simulink model "io305"  (Simulink 6.0)
settings: Solver=ode5  StartTime=0.0  StopTime=5  RelTol=1e-3
libraries: xpcdiamondlib x2
settings Model: Creator=ekbas  LastModifiedBy=ekbas  ExtModeArmWhenConnect=off  BufferReuse=off  ProdHWDeviceType=Specified
settings DataIOCC: SaveFormat=Structure  SignalLoggingName=sigsOut
settings OptimizationCC: OptimizeBlockIOStorage=off  BufferReuse=off  LocalBlockOutputs=off
settings DebuggingCC: CheckExecutionContextPreStartOutputMsg=on  CheckExecutionContextRuntimeOutputMsg=on  SolverPrmCheckMsg=none
settings HardwareCC: ProdHWDeviceType=Specified  TargetHWDeviceType=32-bit Generic  ProdEqTarget=off
settings RTWCC: SystemTargetFile=xpctarget.tlc  TemplateMakefile=xpc_default_tmf  Description=xPC Target  ProcessScript=xpctarget_make_rtw_hook
settings xpcTargetCC: TargetFcnLib=ansi_tfl_tmw.mat  GenFloatMathFcnCalls=ANSI_C  ModelReferenceCompliant=off  LifeSpan=inf
settings SFSimCC: SFSimApplyToAllLibs=on  SFSimBuildMode=Incremental

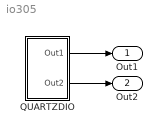
== system io305 ==
  QUARTZDIO : Subsystem  PropExecContextAcrossSSBoundary=on
  Out1 : Outport
  Out2 : Outport  Port=2
  wires:
  QUARTZDIO/1(Out1) -> Out1/1
  QUARTZDIO/2(Out2) -> Out2/1

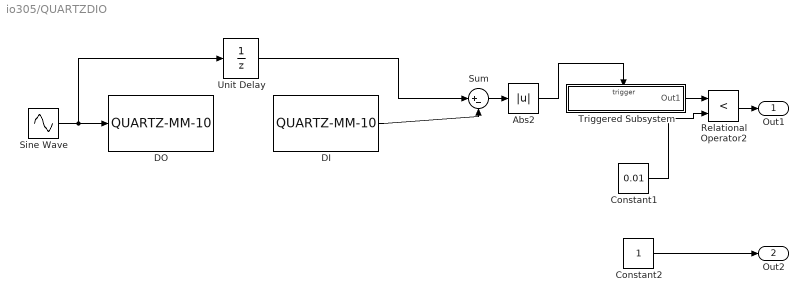
== system io305/QUARTZDIO ==
  Abs2 : Abs  SaturateOnIntegerOverflow=on
  Constant1 : Constant  Value=0.01
  Constant2 : Constant
  DI : xpcdiamondlib/Digital Input/QUARTZ-MM-10   channel=[1]  ts=0.001  baseAddressIn=0x300
  DO : xpcdiamondlib/Digital Output/QUARTZ-MM-10   channel=[3]  ts=0.001  baseAddressIn=0x300
  Relational Operator2 : RelationalOperator  Operator=<
  Sine Wave : Sin  Frequency=5  SampleTime=0.001
  Sum : Sum  Inputs=|+-  SaturateOnIntegerOverflow=on
  Triggered Subsystem : Subsystem  TreatAsAtomicUnit=on  PropExecContextAcrossSSBoundary=on
  Unit Delay : UnitDelay  SampleTime=-1
  Out1 : Outport
  Out2 : Outport  Port=2
  wires:
  Sum/1 -> Abs2/1
  Relational Operator2/1 -> Out1/1
  Sine Wave/1 -> DO/1, Unit Delay/1
  DI/1 -> Sum/2
  Constant2/1 -> Out2/1
  Unit Delay/1 -> Sum/1
  Abs2/1 -> Triggered Subsystem/Trigger
  Triggered Subsystem/1(Out1) -> Relational Operator2/1
  Constant1/1 -> Relational Operator2/2

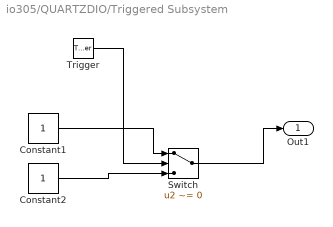
== system io305/QUARTZDIO/Triggered Subsystem ==
  Trigger : TriggerPort  ShowOutputPort=on
  Constant1 : Constant  OutDataTypeMode=double
  Constant2 : Constant  OutDataTypeMode=double
  Switch : Switch  Criteria=u2 ~= 0  InputSameDT=on
  Out1 : Outport
  wires:
  Constant2/1 -> Switch/3
  Constant1/1 -> Switch/1
  Switch/1 -> Out1/1
  Trigger/1 -> Switch/2
